simulink model "model_real"  (R2015a)
settings: Solver=ode3  StartTime=0.0  StopTime=Tmax  RelTol=1e-3
values from neighbouring files (symbols this model uses):
  A = [3.29698189006 1 0 0 -4.20791026518 0 1 0 2.48348543348 0 0 1 ... (16 elements, 4x4)]    [end_of_class.mat]    (also in log_observer_test.mat; parameters.mat)
  B = [1 0 0 0]    [end_of_class.mat]    (also in log_observer_test.mat; parameters.mat)
  C = [-0.0495309545297 0.081302844811 0.0308276179144 0]    [end_of_class.mat]    (also in log_observer_test.mat; parameters.mat)
  K = dlqr(A, B, Q, R)    [compute_gain.m]    (also in end_of_class.mat = [0.679089360081 -1.41789247675 1.07430486636 -0.291654825833; log_observer_test.mat = [0.679089360081 -1.41789247675 1.07430486636 -0.291654825833)
  Ke = -3.922    [end_of_class.mat]    (also in log_observer_test.mat)
  Kp = 34.453    [end_of_class.mat]    (also in log_observer_test.mat)
  M = dlqe(A, G, C, Qw, Rw)    [compute_gain.m]    (also in end_of_class.mat = [46.1937797554 31.7894394899 18.6722805315 9.22195693924]; log_observer_test.mat = [13.0934534825 11.0057014889 8.5354108434 5.97963050629])
  Nbar = Nu+K*Nx    [compute_gain.m]    (also in end_of_class.mat = 0.700435596375; log_observer_test.mat = 0.700435596375)
  T = 0.02    [end_of_class.mat]    (also in gera_signals.m; log_observer_test.mat)
undefined symbols (not defined in the file or in its folder): MIO, National_Instruments, PCI
libraries: sldrtlib x2
settings Model: SimulationMode=external  ExtModeTrigDuration=20000  Creator=alunos  LastModifiedBy=alunos
settings DataIOCC: LimitDataPoints=off
settings HardwareCC: ProdIntDivRoundTo=Zero  ProdEndianess=LittleEndian  ProdHWDeviceType=Intel->x86/Pentium  TargetIntDivRoundTo=Zero  TargetEndianess=LittleEndian  TargetHWDeviceType=Intel->x86/Pentium
settings RTWCC: SystemTargetFile=rtwin.tlc  TemplateMakefile=rtwin.tmf  Description=Simulink Desktop Real-Time  RTWCompilerOptimization=on
settings CodeAppCC: MaxIdLength=95
settings RTWinTargetCC: TargetPreCompLibLocation=C:\Program Files\MATLAB\R2015a\toolbox\sldrt\lib\win32

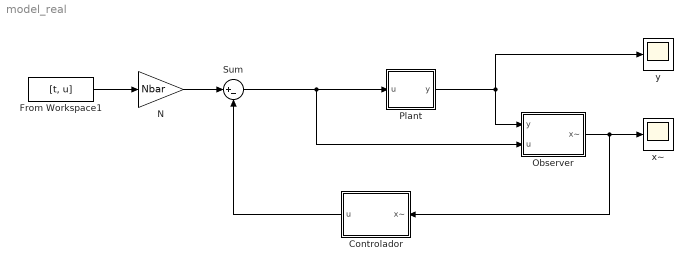
== system model_real ==
  Controlador : Subsystem
  From Workspace1 : FromWorkspace  VariableName=[t, u]  SampleTime=T
  N : Gain  Gain=Nbar
  Observer : Subsystem
  Plant : Subsystem
  Sum : Sum  Inputs=|+-
  x~ : Scope
      settings: TimeRange=20  YMin=-1000  YMax=0  SaveName=ScopeData3
  y : Scope
      settings: TimeRange=20  YMin=-1000  YMax=0
  wires:
  Plant/1(y) -> Observer/1(y), y/1
  Observer/1(x~) -> Controlador/1(x~), x~/1
  Sum/1 -> Observer/2(u), Plant/1(u)
  N/1 -> Sum/1
  From Workspace1/1 -> N/1
  Controlador/1(u) -> Sum/2

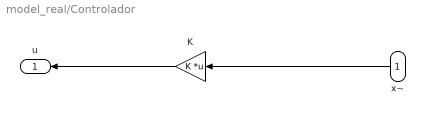
== system model_real/Controlador ==
  x~ : Inport
  K : Gain  Gain=K  Multiplication=Matrix(K*u)
  u : Outport
  wires:
  K/1 -> u/1
  x~/1 -> K/1

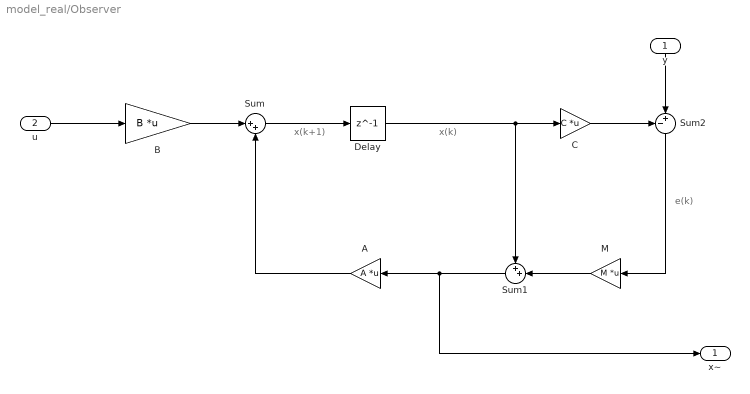
== system model_real/Observer ==
  note: e(k)
  note: x(k)
  note: x(k+1)
  y : Inport  PortDimensions=1
  u : Inport  Port=2
  A : Gain  Gain=A  Multiplication=Matrix(K*u)
  B : Gain  Gain=B  Multiplication=Matrix(K*u) (u vector)
  C : Gain  Gain=C  Multiplication=Matrix(K*u)
  Delay : Delay  DelayLength=1  InitialCondition=[0;0;0;0]
  M : Gain  Gain=M  Multiplication=Matrix(K*u) (u vector)
  Sum : Sum  Inputs=|++
  Sum1 : Sum  Inputs=++|
  Sum2 : Sum  Inputs=-+|
  x~ : Outport  PortDimensions=[4,1]
  wires:
  Sum/1 -> Delay/1
  C/1 -> Sum2/1
  Sum2/1 -> M/1
  Delay/1 -> C/1, Sum1/1
  M/1 -> Sum1/2
  A/1 -> Sum/2
  y/1 -> Sum2/2
  u/1 -> B/1
  Sum1/1 -> x~/1, A/1
  B/1 -> Sum/1

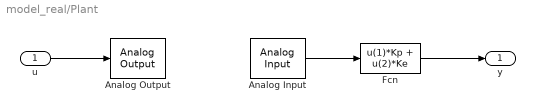
== system model_real/Plant ==
  u : Inport
  Analog Input : sldrtlib/Analog Input  SampleTime=T  MaxMissedTicks=10  ShowMissedTicks=off  YieldWhenWaiting=off  DrvName=National_Instruments/PCI-MIO-16E-4  DrvAddress=4294967295  DrvOptions=[0 0 0 0 0 0]  Channels=1:3  RangeMode=1  VoltRange=1  DataType=1
      settings: AttributesFormatString=National Instruments\nPCI-MIO-16E-4 [auto]
  Analog Output : sldrtlib/Analog Output  SampleTime=T  MaxMissedTicks=10  ShowMissedTicks=off  YieldWhenWaiting=off  DrvName=National_Instruments/PCI-MIO-16E-4  DrvAddress=4294967295  DrvOptions=[0 0 0 0 0 0]  Channels=1  RangeMode=1  VoltRange=1  InitialValue=0  FinalValue=0
      settings: AttributesFormatString=National Instruments\nPCI-MIO-16E-4 [auto]
  Fcn : Fcn  Expr=u(1)*Kp + u(2)*Ke
  y : Outport
  wires:
  Analog Input/1 -> Fcn/1
  u/1 -> Analog Output/1
  Fcn/1 -> y/1
